simulink model "blinker"  (R2015b)
settings: Solver=VariableStepAuto  StartTime=0.0  StopTime=inf  RelTol=1e-3
settings Model: Creator=scco1019  LastModifiedBy=scco1019

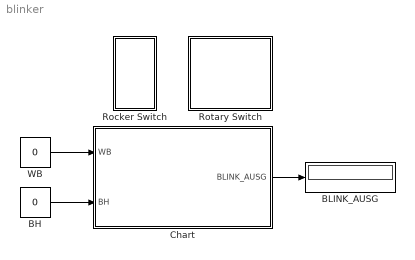
== system blinker ==
  BH : Constant  Value=0
  "BLINK_AUSG " : Display
  Chart : Stateflow chart  TreatAsAtomicUnit=on
  Rocker Switch : Subsystem  DialogController=hmiCreateDDGDialog  IsWebBlock=on  mask(MWDashboardBlock){webBlockId=0bcaf0f6-323e-4941-add3-d349799d6edb, webBlockType=rockerswitch, ShowInLibBrowser=on, ShowInitialText=on, HMISrcModelName=blinker}
      mask prompts: webBlockId "WebBlock Id"; webBlockType "WebBlock Type"; HMISrcModelName "Source Model"
      mask Help: helpview([docroot '/mapfiles/simulink.map'], 'hmi_rocker_switch')
      mask Display:
      | if strcmp(get_param(bdroot(gcb),'BlockDiagramType'), 'library')
      |     image([(matlabroot) '/toolbox/simulink/hmi/icons/RockerSwitch.png']);
      | end
  Rotary Switch : Subsystem  DialogController=hmiCreateDDGDialog  IsWebBlock=on  mask(MWDashboardBlock){webBlockId=c0fe2a19-d1fa-49c2-b61f-8e57bf1be38a, webBlockType=discreteknob, ShowInLibBrowser=on, ShowInitialText=on, HMISrcModelName=blinker}
      mask prompts: webBlockId "WebBlock Id"; webBlockType "WebBlock Type"; HMISrcModelName "Source Model"
      mask Help: helpview([docroot '/mapfiles/simulink.map'], 'hmi_rotary_switch')
      mask Display:
      | model = bdroot(gcb);
      | if strcmp(get_param(model,'BlockDiagramType'), 'library')
      |     image([(matlabroot) '/toolbox/simulink/hmi/icons/DiscreteKnob.png']);
      | end
  WB : Constant  Value=0
  wires:
  WB/1 -> Chart/1(WB)
  BH/1 -> Chart/2(BH)
  Chart/1(BLINK_AUSG) -> "BLINK_AUSG "/1

== system blinker/Rocker Switch ==

== system blinker/Rotary Switch ==

== stateflow chart blinker/Chart ==
  state AUS/
    entry: BLINK_AUSG=0;
    local=0;
  state LINKS/
    entry: BLINK_AUSG=1;
  state RECHTS/
    entry: BLINK_AUSG=2;
  state WB_AN/
    entry: BLINK_AUSG=3;
  (default) -> AUS
  RECHTS -> RECHTS [order 3] : [WB==0]
      | {local=1}
  LINKS -> LINKS [order 3] : [WB==0]
      | {local=1}
  LINKS -> LINKS [order 4]
  RECHTS -> RECHTS [order 4]
  AUS -> RECHTS [order 1] : [BH==2]
      | {local=1}
  AUS -> LINKS [order 3] : [BH==1]
      | {local=1}
  RECHTS -> AUS [order 2] : [BH~=2]
      | {local=0}
  LINKS -> AUS [order 2] : [BH~=1]
      | {local=0}
  LINKS -> WB_AN [order 1] : [WB==1&&local==1]
      | {local=3}
  WB_AN -> LINKS [order 1] : [BH==1&&local==2]
  WB_AN -> RECHTS [order 2] : [BH==2&&local==2]
  RECHTS -> WB_AN [order 1] : [WB==1&&local==1]
      | {local=3}
  WB_AN -> AUS [order 3] : [WB==0]
      | {local=0}
  AUS -> WB_AN [order 2] : [WB==1]
      | {local=2}
  WB_AN -> WB_AN [order 4] : [BH==0]
      | {local=2}
  WB_AN -> WB_AN [order 5]
  data: WB input; BH input; BLINK_AUSG output; local local
